simulink model "RC_Circuit"  (R2023a)
settings: Solver=VariableStepAuto  StartTime=0.0  StopTime=10.0  RelTol=1e-3
values from neighbouring files (symbols this model uses):
  C = 5    [script.m]
  R = 10    [script.m]
settings Model: Creator=eslam  LastModifiedBy=eslam

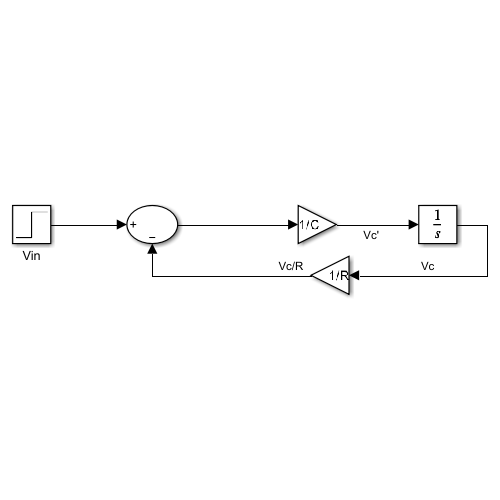
[thumbnail: Simulink's stored preview of the top-level diagram]
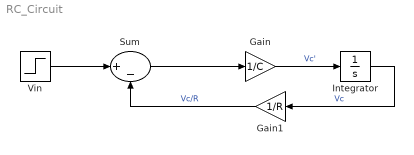
== system RC_Circuit ==
  Gain : Gain  Gain=1/C
  Gain1 : Gain  Gain=1/R
  Integrator : Integrator
  Sum : Sum  Inputs=|+-
  Vin : Step  SampleTime=0
  wires:
  Vin/1 -> Sum/1
  Sum/1 -> Gain/1
  Gain/1 -> Integrator/1  "Vc'"
  Integrator/1 -> Gain1/1  "Vc"
  Gain1/1 -> Sum/2  "Vc/R"
